simulink model "Controller"  (R2025b)
settings: Solver=ode1  StartTime=0.0  StopTime=10  FixedStep=0.001  RelTol=1e-3
values from neighbouring files (symbols this model uses):
  ISCS_Tu = diag([u_alpha_nom, du_ign_nom])    [LQGI.m]    (also in LQGI_test.m)
  ISCS_Ty = omega_e_nom    [LQGI.m]    (also in LQGI_test.m)
  ISCSAd = sysD.A    [LQGI.m]
  ISCSBd = sysD.B    [LQGI.m]
  ISCSCd = sysD.C    [LQGI.m]
settings Model: Creator=khanh  LastModifiedBy=khanh

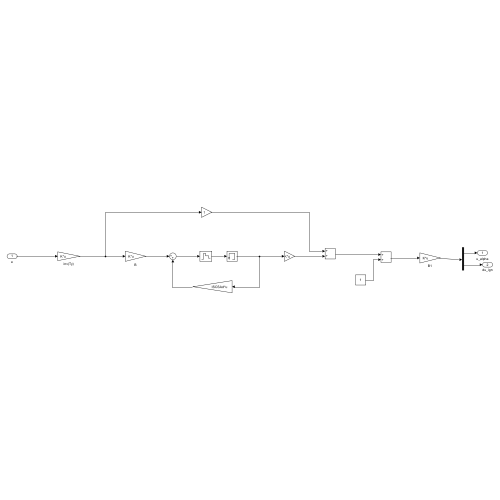
[thumbnail: Simulink's stored preview of the top-level diagram]
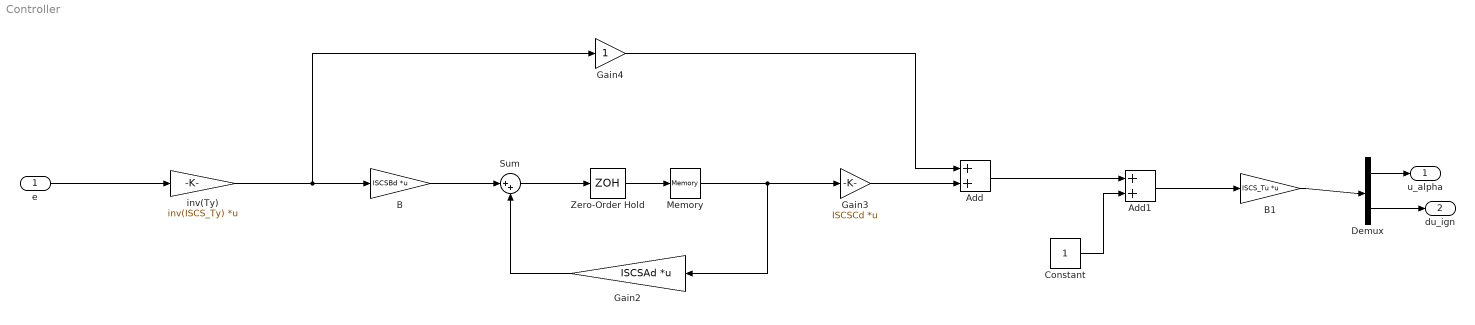
== system Controller ==
  e : Inport
  Add : Sum
  Add1 : Sum
  B : Gain  Gain=ISCSBd  Multiplication=Matrix(K*u)
  B1 : Gain  Gain=ISCS_Tu  Multiplication=Matrix(K*u)
  Constant : Constant
  Demux : Demux  Outputs=2
  Gain2 : Gain  Gain=ISCSAd  Multiplication=Matrix(K*u)
  Gain3 : Gain  Gain=ISCSCd  Multiplication=Matrix(K*u)
  Gain4 : Gain
  Memory : Memory
  Sum : Sum  Inputs=|++
  Zero-Order Hold : ZeroOrderHold  SampleTime=0.001
  inv(Ty) : Gain  Gain=inv(ISCS_Ty)  Multiplication=Matrix(K*u)
  u_alpha : Outport
  du_ign : Outport  Port=2
  wires:
  e/1 -> inv(Ty)/1
  inv(Ty)/1 -> Gain4/1, B/1
  B/1 -> Sum/1
  Sum/1 -> Zero-Order Hold/1
  Zero-Order Hold/1 -> Memory/1
  Memory/1 -> Gain3/1, Gain2/1
  Gain2/1 -> Sum/2
  Gain3/1 -> Add/2
  Gain4/1 -> Add/1
  Add/1 -> Add1/1
  Constant/1 -> Add1/2
  Add1/1 -> B1/1
  B1/1 -> Demux/1
  Demux/1 -> u_alpha/1
  Demux/2 -> du_ign/1
